simulink model "DCV_tester2"  (R2024b)
settings: Solver=VariableStepAuto  StartTime=0.0  StopTime=11.5  RelTol=1e-3
settings Model: Creator=Emil  LastModifiedBy=Emil

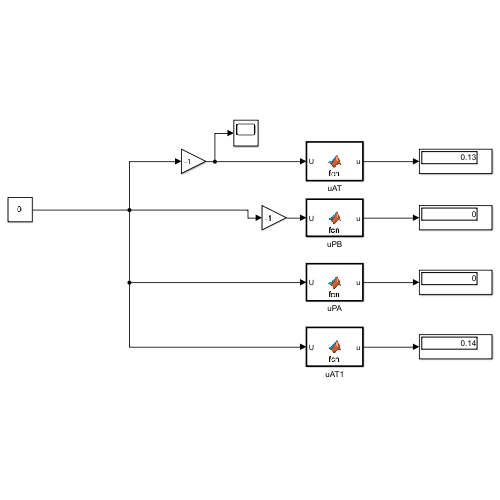
[thumbnail: Simulink's stored preview of the top-level diagram]
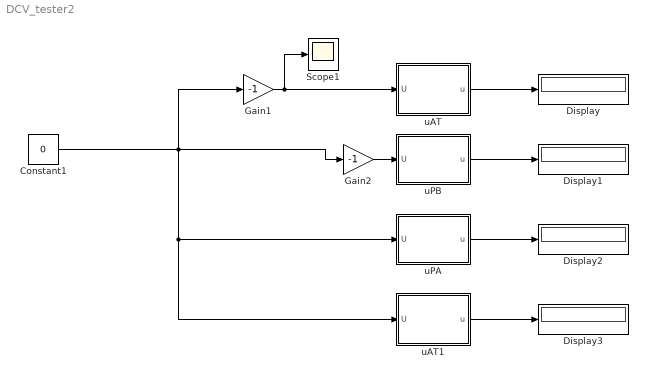
== system DCV_tester2 ==
  Constant1 : Constant  Value=0
  Display{,1..3} (4 alike) : Display
  Gain1 : Gain  Gain=-1
  Gain2 : Gain  Gain=-1
  Scope1 : Scope
  uAT : MATLAB Function  TreatAsAtomicUnit=on
  uAT1 : MATLAB Function  TreatAsAtomicUnit=on
  uPA : MATLAB Function  TreatAsAtomicUnit=on
  uPB : MATLAB Function  TreatAsAtomicUnit=on
  wires:
  Constant1/1 -> uAT1/1(U), uPA/1(U), Gain2/1, Gain1/1
  uAT/1(u) -> Display/1
  uPB/1(u) -> Display1/1
  Gain2/1 -> uPB/1(U)
  uPA/1(u) -> Display2/1
  Gain1/1 -> uAT/1(U), Scope1/1
  uAT1/1(u) -> Display3/1

== matlab function DCV_tester2/uAT1 ==
  data: U input; u output
function u = fcn(U)
if U < -0.13
    u=0;
elseif U <= 0
    u = 0.14-abs(U);
elseif U <= 0.14
    u = 0.14;
elseif U >0.14
    u= (U-0.14)/(1-0.14)+0.14;
else
    u = 0;
end
% u = u+0.15;

== matlab function DCV_tester2/uPB ==
  data: U input; u output
function u = fcn(U)
if U < 0.13
    u = 0;
elseif U >=0.13
    u= (U-0.13)/(1-0.13);
else
    u = 0;
end

== matlab function DCV_tester2/uAT ==
  data: U input; u output
function u = fcn(U)
if U < -0.14
    u=0;
elseif U <= 0
    u = 0.13-abs(U);
elseif U <= 0.13
    u = 0.13;
elseif U >0.13
    u= (U-0.13)/(1-0.13)+0.13;
else
    u = 0;
end
% u = u+0.15;

== matlab function DCV_tester2/uPA ==
  data: U input; u output
function u = fcn(U)
if U < 0.14
    u = 0;
elseif U >=0.14
    u= (U-0.14)/(1-0.14);
else
    u = 0;
end
